simulink model "trav_techo_PLANT"  (R2022a)
settings: Solver=VariableStepAuto  StartTime=0.0  StopTime=100.0  RelTol=1e-3
undefined symbols (not defined in the file or in its folder): fix_constt, JLrtt, JMrtt, Kktt, Kvtt
libraries: slctrlblks x1
settings Model: Creator=ohadformanair  LastModifiedBy=ohadformanair
settings SolverCC: ZeroCrossAlgorithm=Adaptive
settings DebuggingCC: IgnoredZcDiagnostic=none

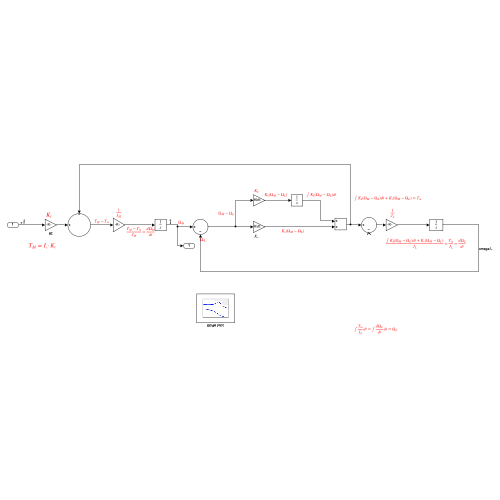
[thumbnail: Simulink's stored preview of the top-level diagram]
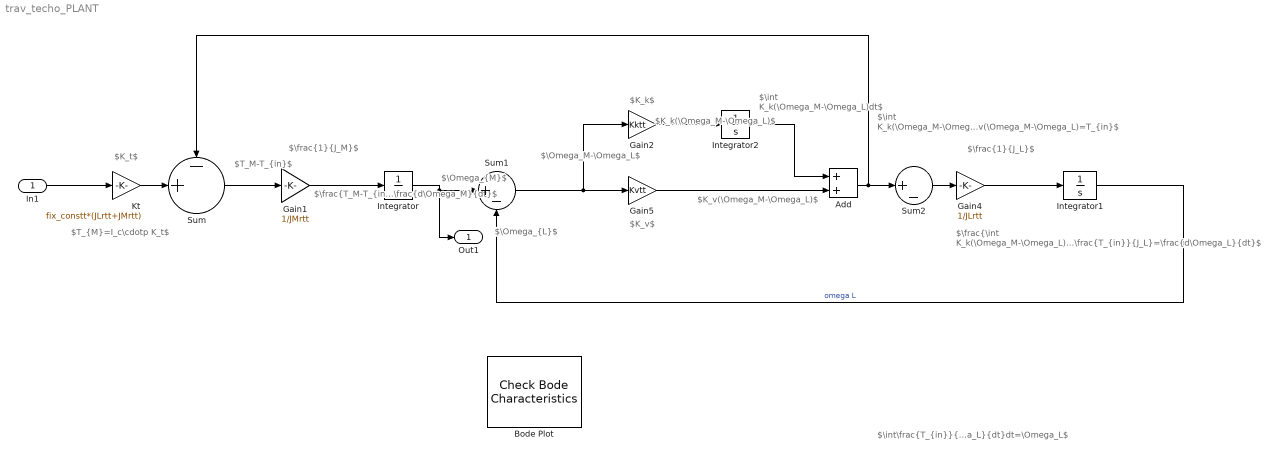
== system trav_techo_PLANT ==
  note: $\frac{T_M-T_{in}}{J_M}=\frac{d\Omega_M}{dt}$
  note: $K_v(\Omega_M-\Omega_L)$
  note: $\frac{\int K_k(\Omega_M-\Omega_L)dt+K_v(\Omega_M-\Omega_L)}{J_L}=\frac{T_{in}}{J_L}=\frac{d\Omega_L}{dt}$
  note: $\int K_k(\Omega_M-\Omega_L)dt$
  note: $T_M-T_{in}$
  note: $K_t$
  note: $T_{M}=I_c\cdotp K_t$
  note: $K_k$
  note: $\int\frac{T_{in}}{J_L}dt=\int\frac{d\Omega_L}{dt}dt=\Omega_L$
  note: $\int K_k(\Omega_M-\Omega_L)dt+K_v(\Omega_M-\Omega_L)=T_{in}$
  note: $\frac{1}{J_L}$
  note: $\Omega_{M}$
  note: $K_k(\Omega_M-\Omega_L)$
  note: $\frac{1}{J_M}$
  note: $K_v$
  note: $\Omega_M-\Omega_L$
  note: $\Omega_{L}$
  In1 : Inport
  Add : Sum
  Bode Plot : slctrlblks/Model Verification/Check Bode  Characteristics  InstantiateOnLoad=on  SaveOperatingPoints=off  LinearizationIOs={'/In1', 1, 'in', 'off', '';'/Integrator', 1, 'out', 'off', ''}  LinearizeAt=SnapshotTimes  SnapshotTimes=[0]  TriggerType=rising  SampleTime=auto  RateConversionMethod=zoh  PreWarpFreq=10  UseExactDelayModel=off  UseFullBlockNameLabels=off  UseBusSignalLabels=off  enabled=on  stopWhenAssertionFail=off  export=off  ViewDlgPos=[100 130 767 460]  OpenViewOnLoad=off  LaunchViewOnOpen=off  FrequencyUnits=Hz  MagnitudeUnits=dB  PhaseUnits=deg  TimeUnits=seconds  EnableUpperBound=off  UpperBoundFrequencies=[]  UpperBoundMagnitudes=[]  EnableLowerBound=off  LowerBoundFrequencies=[]  LowerBoundMagnitudes=[]
  Gain1 : Gain  Gain=1/JMrtt
  Gain2 : Gain  Gain=Kktt
  Gain4 : Gain  Gain=1/JLrtt
  Gain5 : Gain  Gain=Kvtt
  Integrator : Integrator
  Integrator1 : Integrator
  Integrator2 : Integrator
  Kt : Gain  Gain=fix_constt*(JLrtt+JMrtt)
  Sum : Sum  Inputs=-+|
  Sum1 : Sum  Inputs=|+-
  Sum2 : Sum  Inputs=|+-
  Out1 : Outport
  wires:
  Integrator/1 -> Out1/1, Sum1/1
  Gain1/1 -> Integrator/1
  Gain2/1 -> Integrator2/1
  Gain5/1 -> Add/2
  Integrator2/1 -> Add/1
  Gain4/1 -> Integrator1/1
  Add/1 -> Sum2/1, Sum/1
  Sum1/1 -> Gain5/1, Gain2/1
  Integrator1/1 -> Sum1/2  "omega L"
  Sum/1 -> Gain1/1
  Kt/1 -> Sum/2
  Sum2/1 -> Gain4/1
  In1/1 -> Kt/1
